simulink model "schema"  (R2015a)
settings: Solver=ode3  StartTime=0.0  StopTime=inf  FixedStep=1e-3  RelTol=1e-3
values from neighbouring files (symbols this model uses):
  conversion_V2mm = 17.8/(3540-260)    (= 0.00542682926829)    [main.m]
  L_vect = sqrt((V_vect./I_vect).^2 - R^2)./31.4    [main.m]
  N = 2*860    (= 1720)    [main.m]
  parameter = [m,R,N,Lb,Pb,d0,u0,cr,x0,Lfe,ur,As]    [main.m]
  x_vect = fliplr([0,1.8,2.4,6.56,9.99,14.04,17.8])    [main.m]
undefined symbols (not defined in the file or in its folder): fdesignblkfcn, gcbh
libraries: PoliArd x5, simulink x3
settings Model: ExtModeTrigDuration=2  Creator=User  LastModifiedBy=User
settings OptimizationCC: OptimizeModelRefInitCode=on  LifeSpan=1
settings DebuggingCC: UnderspecifiedInitializationDetection=Classic  MergeDetectMultiDrivingBlocksExec=none
settings HardwareCC: ProdLargestAtomicInteger=Long  ProdLargestAtomicFloat=Double  ProdEndianess=LittleEndian  ProdHWDeviceType=ARM Compatible->ARM Cortex
settings RTWCC: SystemTargetFile=realtime.tlc  GenerateMakefile=off  TemplateMakefile=realtime.tmf  Description=Run on Target Hardware  RTWVerbose=off
settings ERTTargetCC: CombineOutputUpdateFcns=off  ExtModeTransport=3  ExtModeMexFile=ext_serial_win32_comm_rtt  ExtModeMexArgs=0 1 9600  ERTSrcFileBannerTemplate=realtime_code_template.cgt  ERTHdrFileBannerTemplate=realtime_code_template.cgt  ERTDataSrcFileTemplate=realtime_code_template.cgt  ERTDataHdrFileTemplate=realtime_code_template.cgt  ERTCustomFileTemplate=realtime_file_process.tlc

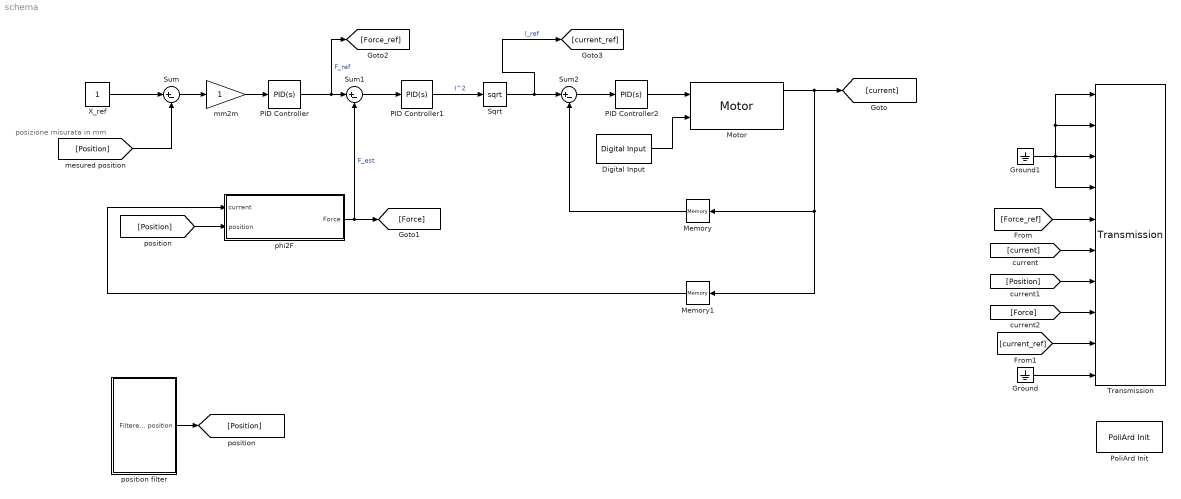
== system schema ==
  note: posizione
      | misurata
      | in mm
  Digital Input : PoliArd/Digital Input  DI_pin=2  DIsample=-1
  Ground : Ground
  Ground1 : Ground
  Memory : Memory
  Memory1 : Memory
  Motor : PoliArd/Motor  MotorID=2  DC_bus_mask=24  dt_mot=-1
  PID Controller : simulink/Continuous/PID Controller  Controller=PID  TimeDomain=Continuous-time  SampleTime=-1  IntegratorMethod=Forward Euler  FilterMethod=Forward Euler  Form=Parallel  UseFilter=on  ControllerParametersSource=internal  P=1000  I=0  D=0  N=100  InitialConditionSource=internal  InitialConditionForIntegrator=0  InitialConditionForFilter=0  ExternalReset=none  LimitOutput=off  UpperSaturationLimit=inf  LowerSaturationLimit=-inf  LinearizeAsGain=on  AntiWindupMode=none  Kb=1  TrackingMode=off  Kt=1  PParamMin=[]  PParamMax=[]  IParamMin=[]  IParamMax=[]  DParamMin=[]  DParamMax=[]  NParamMin=[]  NParamMax=[]  KbParamMin=[]  KbParamMax=[]  KtParamMin=[]  KtParamMax=[]  POutMin=[]  POutMax=[]  IOutMin=[]  IOutMax=[]  DOutMin=[]  DOutMax=[]  NOutMin=[]  NOutMax=[]  KbOutMin=[]  KbOutMax=[]  KtOutMin=[]  KtOutMax=[]  IntegratorOutMin=[]  IntegratorOutMax=[]  FilterOutMin=[]  FilterOutMax=[]  SumOutMin=[]  SumOutMax=[]  SumI1OutMin=[]  SumI1OutMax=[]  SumI2OutMin=[]  SumI2OutMax=[]  SumI3OutMin=[]  SumI3OutMax=[]  SumDOutMin=[]  SumDOutMax=[]  SaturationOutMin=[]  SaturationOutMax=[]  IntegratorContinuousStateAttributes=''  IntegratorStateMustResolveToSignalObject=off  IntegratorRTWStateStorageClass=Auto  FilterContinuousStateAttributes=''  FilterStateMustResolveToSignalObject=off  FilterRTWStateStorageClass=Auto  DifferentiatorICPrevScaledInput=0  DifferentiatorOutMin=[]  DifferentiatorOutMax=[]
  PID Controller1 : simulink/Continuous/PID Controller  Controller=PID  TimeDomain=Continuous-time  SampleTime=-1  IntegratorMethod=Forward Euler  FilterMethod=Forward Euler  Form=Parallel  UseFilter=on  ControllerParametersSource=internal  P=10000  I=0  D=0  N=100  InitialConditionSource=internal  InitialConditionForIntegrator=0  InitialConditionForFilter=0  ExternalReset=none  LimitOutput=off  UpperSaturationLimit=inf  LowerSaturationLimit=-inf  LinearizeAsGain=on  AntiWindupMode=none  Kb=1  TrackingMode=off  Kt=1  PParamMin=[]  PParamMax=[]  IParamMin=[]  IParamMax=[]  DParamMin=[]  DParamMax=[]  NParamMin=[]  NParamMax=[]  KbParamMin=[]  KbParamMax=[]  KtParamMin=[]  KtParamMax=[]  POutMin=[]  POutMax=[]  IOutMin=[]  IOutMax=[]  DOutMin=[]  DOutMax=[]  NOutMin=[]  NOutMax=[]  KbOutMin=[]  KbOutMax=[]  KtOutMin=[]  KtOutMax=[]  IntegratorOutMin=[]  IntegratorOutMax=[]  FilterOutMin=[]  FilterOutMax=[]  SumOutMin=[]  SumOutMax=[]  SumI1OutMin=[]  SumI1OutMax=[]  SumI2OutMin=[]  SumI2OutMax=[]  SumI3OutMin=[]  SumI3OutMax=[]  SumDOutMin=[]  SumDOutMax=[]  SaturationOutMin=[]  SaturationOutMax=[]  IntegratorContinuousStateAttributes=''  IntegratorStateMustResolveToSignalObject=off  IntegratorRTWStateStorageClass=Auto  FilterContinuousStateAttributes=''  FilterStateMustResolveToSignalObject=off  FilterRTWStateStorageClass=Auto  DifferentiatorICPrevScaledInput=0  DifferentiatorOutMin=[]  DifferentiatorOutMax=[]
  PID Controller2 : simulink/Continuous/PID Controller  Controller=PID  TimeDomain=Continuous-time  SampleTime=-1  IntegratorMethod=Forward Euler  FilterMethod=Forward Euler  Form=Parallel  UseFilter=on  ControllerParametersSource=internal  P=1  I=1  D=0  N=100  InitialConditionSource=internal  InitialConditionForIntegrator=0  InitialConditionForFilter=0  ExternalReset=none  LimitOutput=off  UpperSaturationLimit=inf  LowerSaturationLimit=-inf  LinearizeAsGain=on  AntiWindupMode=none  Kb=1  TrackingMode=off  Kt=1  PParamMin=[]  PParamMax=[]  IParamMin=[]  IParamMax=[]  DParamMin=[]  DParamMax=[]  NParamMin=[]  NParamMax=[]  KbParamMin=[]  KbParamMax=[]  KtParamMin=[]  KtParamMax=[]  POutMin=[]  POutMax=[]  IOutMin=[]  IOutMax=[]  DOutMin=[]  DOutMax=[]  NOutMin=[]  NOutMax=[]  KbOutMin=[]  KbOutMax=[]  KtOutMin=[]  KtOutMax=[]  IntegratorOutMin=[]  IntegratorOutMax=[]  FilterOutMin=[]  FilterOutMax=[]  SumOutMin=[]  SumOutMax=[]  SumI1OutMin=[]  SumI1OutMax=[]  SumI2OutMin=[]  SumI2OutMax=[]  SumI3OutMin=[]  SumI3OutMax=[]  SumDOutMin=[]  SumDOutMax=[]  SaturationOutMin=[]  SaturationOutMax=[]  IntegratorContinuousStateAttributes=''  IntegratorStateMustResolveToSignalObject=off  IntegratorRTWStateStorageClass=Auto  FilterContinuousStateAttributes=''  FilterStateMustResolveToSignalObject=off  FilterRTWStateStorageClass=Auto  DifferentiatorICPrevScaledInput=0  DifferentiatorOutMin=[]  DifferentiatorOutMax=[]
  PoliArd Init : PoliArd/PoliArd Init
  Sqrt : Sqrt  SaturateOnIntegerOverflow=on
  Sum : Sum  Inputs=|+-
  Sum1 : Sum  Inputs=|+-
  Sum2 : Sum  Inputs=|+-
  Transmission : PoliArd/Transmission  sample_freq=100  sig_to_send=6
  X_ref : Constant
  mm2m : Gain
  phi2F : Subsystem
  position filter : Subsystem
  wires:
  Motor/1 -> [current], Memory/1, Memory1/1
  Sum/1 -> mm2m/1
  position filter/1("Filtered position ") -> [Position]
  [Position] -> Sum/2
  [Position] -> phi2F/2(position)
  PID Controller/1 -> [Force_ref], Sum1/1  "F_ref"
  phi2F/1("Force ") -> [Force], Sum1/2  "F_est"
  Sum1/1 -> PID Controller1/1
  PID Controller1/1 -> Sqrt/1  "I^2"
  X_ref/1 -> Sum/1
  Sum2/1 -> PID Controller2/1
  PID Controller2/1 -> Motor/1
  [current] -> Transmission/6
  [Position] -> Transmission/7
  [Force] -> Transmission/8
  Ground/1 -> Transmission/10
  Ground1/1 -> Transmission/4, Transmission/2, Transmission/1, Transmission/3
  Sqrt/1 -> [current_ref], Sum2/1  "I_ref"
  Digital Input/1 -> Motor/2
  Memory/1 -> Sum2/2
  Memory1/1 -> phi2F/1(current)
  mm2m/1 -> PID Controller/1
  [Force_ref] -> Transmission/5
  [current_ref] -> Transmission/9

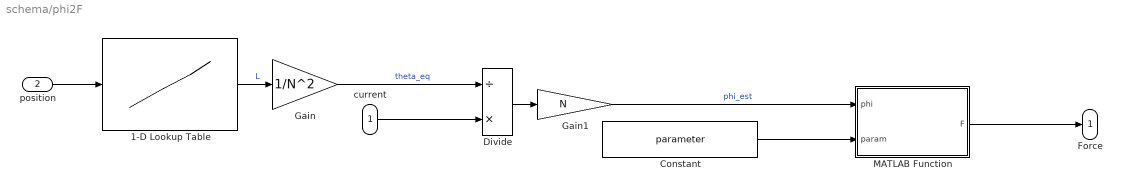
== system schema/phi2F ==
  current : Inport
  position : Inport  Port=2
  1-D Lookup Table : Lookup_n-D  NumberOfTableDimensions=1  BreakpointsForDimension1=L_vect  Table=x_vect  ExtrapMethod=Clip  InternalRulePriority=Speed  RndMeth=Simplest  InputSameDT=on
  Constant : Constant  Value=parameter
  Divide : Product  Inputs=/*
  Gain : Gain  Gain=1/N^2
  Gain1 : Gain  Gain=N
  MATLAB Function : MATLAB Function  TreatAsAtomicUnit=on
  "Force " : Outport
  wires:
  Gain1/1 -> MATLAB Function/1(phi)  "phi_est"
  Divide/1 -> Gain1/1
  1-D Lookup Table/1 -> Gain/1  "L"
  Constant/1 -> MATLAB Function/2(param)
  Gain/1 -> Divide/1  "theta_eq"
  current/1 -> Divide/2
  MATLAB Function/1(F) -> "Force "/1
  position/1 -> 1-D Lookup Table/1

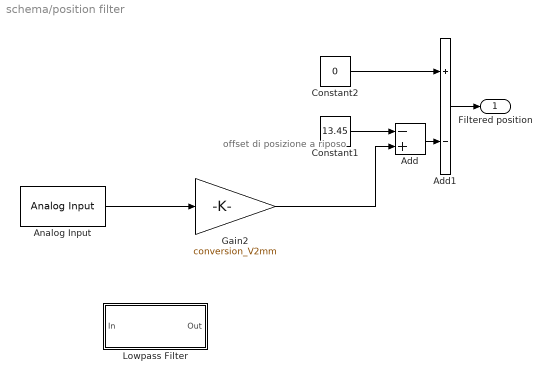
== system schema/position filter ==
  note: offset di posizione a riposo
  Add : Sum  Inputs=-+
  Add1 : Sum  Inputs=+-
  Analog Input : PoliArd/Analog Input  AIpin_mask=2  AIsample=-1
  Constant1 : Constant  Value=13.45
  Constant2 : Constant  Value=0
  Gain2 : Gain  Gain=conversion_V2mm
  Lowpass Filter : Subsystem  DialogController=fdesignblkfcn  InitFcn=fdesignblkfcn(gcbh, {'InitFcn'});  mask(Lowpass Filter){}
      mask help: Design a lowpass filter
      settings: CopyFcn=fdesignblkfcn(gcbh, {'CopyFcn'});
      mask Help: helpview(mapfilelocation('dsp'), 'dsplowpassfilter');
      mask Display: disp('Lowpass')
  "Filtered position " : Outport
  wires:
  Gain2/1 -> Add/2
  Constant2/1 -> Add1/1
  Constant1/1 -> Add/1
  Add1/1 -> "Filtered position "/1
  Add/1 -> Add1/2
  Analog Input/1 -> Gain2/1

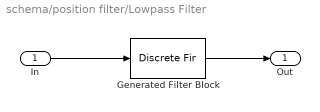
== system schema/position filter/Lowpass Filter ==
  In : Inport
  Generated Filter Block : DiscreteFir  Tag=BlockMethodSubSystem  Coefficients=[-0.096626420854236783 0.24327035766280955 0.68025369464798469 0.24327035766280955 -0.096626420854236783]  InputProcessing=Columns as channels (frame based)
  Out : Outport
  wires:
  In/1 -> Generated Filter Block/1
  Generated Filter Block/1 -> Out/1

== matlab function schema/phi2F/MATLAB Function ==
  data: phi input; F output; param input
function F = fcn(phi,param)
mu0 = param(7,1);
S   = param(12,1);

F = phi^2 / mu0*S;

end
